simulink model "GPS_pll_bak"  (Simulink 6.1)
settings: Solver=ode45  StartTime=0.0  StopTime=1000  RelTol=1e-5
values from neighbouring files (symbols this model uses):
  Ga = 2    [GPS_pll_init.m]    (also in GPS_pll_init_148.m = 0.0625; GPS_pll_init_bak.m = 0.03125)
  Gb = 2    [GPS_pll_init.m]    (also in GPS_pll_init_148.m = 16; GPS_pll_init_bak.m)
  Gdac = 2^-16*5    (= 7.62939453125e-05)    [GPS_pll_init.m]    (also in GPS_pll_init_148.m; GPS_pll_init_bak.m = 5.03540039062e-05)
  Kv = 4e-6    (= 4e-06)    [GPS_pll_init.m]    (also in GPS_pll_init_148.m = 9e-05; GPS_pll_init_bak.m)
  Ts = 1/100e6    (= 1e-08)    [GPS_pll_init.m]    (also in GPS_pll_init_148.m = 6.73400673401e-09; GPS_pll_init_bak.m = 5e-09)
libraries: simulink x1
settings Model: LastModifiedBy=Jens
settings DataIOCC: SignalLoggingName=sigsOut
settings HardwareCC: TargetUnknown=on

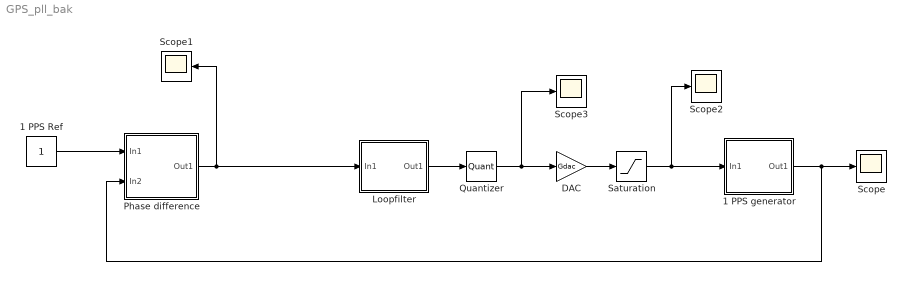
== system GPS_pll_bak ==
  1 PPS Ref : Constant
  1 PPS generator : Subsystem
  DAC : Gain  Gain=Gdac  SaturateOnIntegerOverflow=on
  Loopfilter : Subsystem
  Phase difference : Subsystem
  Quantizer : Quantizer  QuantizationInterval=1
  Saturation : Saturate  UpperLimit=3.3/2  LowerLimit=-3.3/2
  Scope{,1..3} (4 alike) : Scope
      Scope1 settings: SampleInput=on  SampleTime=1
      Scope2 settings: SaveName=ScopeData2  SampleInput=on  SampleTime=1
      Scope3 settings: SaveName=ScopeData3  SampleInput=on  SampleTime=1
  wires:
  1 PPS Ref/1 -> Phase difference/1(In1)
  1 PPS generator/1(Out1) -> Scope/1, Phase difference/2(In2)
  Phase difference/1(Out1) -> Scope1/1, Loopfilter/1(In1)
  DAC/1 -> Saturation/1
  Quantizer/1 -> DAC/1, Scope3/1
  Saturation/1 -> 1 PPS generator/1(In1), Scope2/1
  Loopfilter/1(Out1) -> Quantizer/1

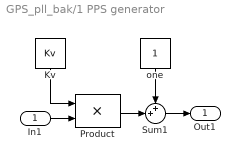
== system GPS_pll_bak/1 PPS generator ==
  In1 : Inport  Port=1  LatchInput=off
  Kv : Constant  Orientation=down  Value=Kv
  Product : Product  SaturateOnIntegerOverflow=on
  Sum1 : Sum  Inputs=++|  SaturateOnIntegerOverflow=on
  one : Constant  Orientation=down
  Out1 : Outport
  wires:
  Kv/1 -> Product/1
  Product/1 -> Sum1/2
  one/1 -> Sum1/1
  Sum1/1 -> Out1/1
  In1/1 -> Product/2

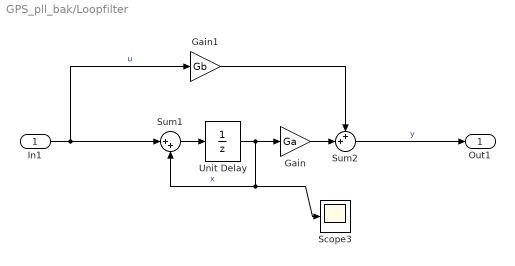
== system GPS_pll_bak/Loopfilter ==
  In1 : Inport  Port=1  LatchInput=off
  Gain : Gain  Gain=Ga  SaturateOnIntegerOverflow=on
  Gain1 : Gain  Gain=Gb  SaturateOnIntegerOverflow=on
  Scope3 : Scope
      settings: SaveName=ScopeData4  SampleInput=on  SampleTime=1
  Sum1 : Sum  Inputs=|++  SaturateOnIntegerOverflow=on
  Sum2 : Sum  Inputs=++|  SaturateOnIntegerOverflow=on
  Unit Delay : UnitDelay
  Out1 : Outport
  wires:
  In1/1 -> Gain1/1, Sum1/1  "u"
  Gain/1 -> Sum2/2
  Gain1/1 -> Sum2/1
  Sum2/1 -> Out1/1  "y"
  Unit Delay/1 -> Gain/1, Sum1/2, Scope3/1  "x"
  Sum1/1 -> Unit Delay/1

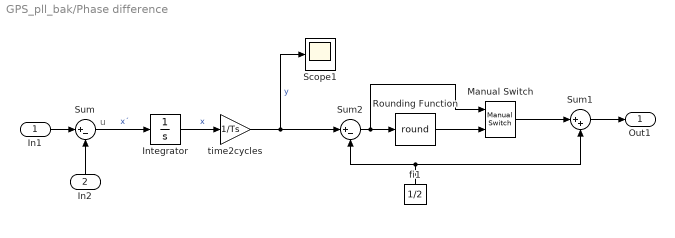
== system GPS_pll_bak/Phase difference ==
  note: u
  In1 : Inport  Port=1  LatchInput=off
  In2 : Inport  Orientation=up  Port=2  LatchInput=off
  Integrator : Integrator  InitialCondition=7000*Ts
  Manual Switch : simulink/Signal Routing/Manual Switch  sw=0  action=0
  Rounding Function : Rounding  Operator=round
  Scope1 : Scope
      settings: SaveName=ScopeData5  SampleInput=on  SampleTime=1
  Sum : Sum  Inputs=|+-  SaturateOnIntegerOverflow=on
  Sum1 : Sum  Inputs=|++  SaturateOnIntegerOverflow=on
  Sum2 : Sum  Inputs=|+-  SaturateOnIntegerOverflow=on
  fi1 : Constant  Orientation=up  Value=1/2
  time2cycles : Gain  Gain=1/Ts  SaturateOnIntegerOverflow=on
  Out1 : Outport
  wires:
  Sum/1 -> Integrator/1  "x´"
  In2/1 -> Sum/2
  Integrator/1 -> time2cycles/1  "x"
  In1/1 -> Sum/1
  fi1/1 -> Sum1/2, Sum2/2
  Sum2/1 -> Manual Switch/1, Rounding Function/1
  Sum1/1 -> Out1/1
  Manual Switch/1 -> Sum1/1
  Rounding Function/1 -> Manual Switch/2
  time2cycles/1 -> Sum2/1, Scope1/1  "y"
